simulink model "regcontrol_model_3ph_old"  (R2018b)
settings: Solver=VariableStepAuto  StartTime=0.0  StopTime=10.0  RelTol=1e-3
values from neighbouring files (symbols this model uses):
  BandWidth = Simulink.Parameter    [start.m]
  BaseVoltage = Simulink.Parameter    [start.m]
  CogenEnabled = false    [regcontrol_emulator.m]    (also in start.m = Simulink.Parameter)
  FPTphase = Simulink.Parameter(FPTphases.DEFAULT)    [regcontrol_emulator.m]    (also in start.m = 1)
  IsReversible = Simulink.Parameter    [start.m]
  LDC_Z = Simulink.Parameter    [start.m]
  MaxTap = 1.10    (= 1.1)    [Transformer.m]
  MinTap = 0.90    (= 0.9)    [Transformer.m]
  PTratio = Simulink.Parameter    [start.m]
  R = 0    [start.m]
  RevBand = Simulink.Parameter    [start.m]
  RevVreg = Simulink.Parameter    [start.m]
  TapLimitPerChange = Simulink.Parameter    [start.m]
  UsingRegulatedBus = Simulink.Parameter    [start.m]
  Vlimit = Simulink.Parameter    [start.m]
  Vreg = Simulink.Parameter    [start.m]
  X = 0    [start.m]
undefined symbols (not defined in the file or in its folder): ControlledTransformerConnection, ControlledTransformerCurrents, ControlledTransformerPowers, ControlledTransformerVoltages, ControlModes, CTRating, IsInverseTime, m, n, NumConductors, NumPhases, PresentTap, RevDelay, revLDC_Z, RevPowerThreshold, revR, revX, TapDelay, TapIncrement, TapWinding, TimeDelay, VTerminal
(part 1 of 4)
settings Model: Creator=Michael Girbino  LastModifiedBy=Michael Girbino
settings DebuggingCC: LibraryContextMissingDiagnostic=none
settings SFSimCC: SimUseLocalCustomCode=off
settings RTWCC: RTWUseLocalCustomCode=off
settings CodeAppCC: StateflowObjectComments=on

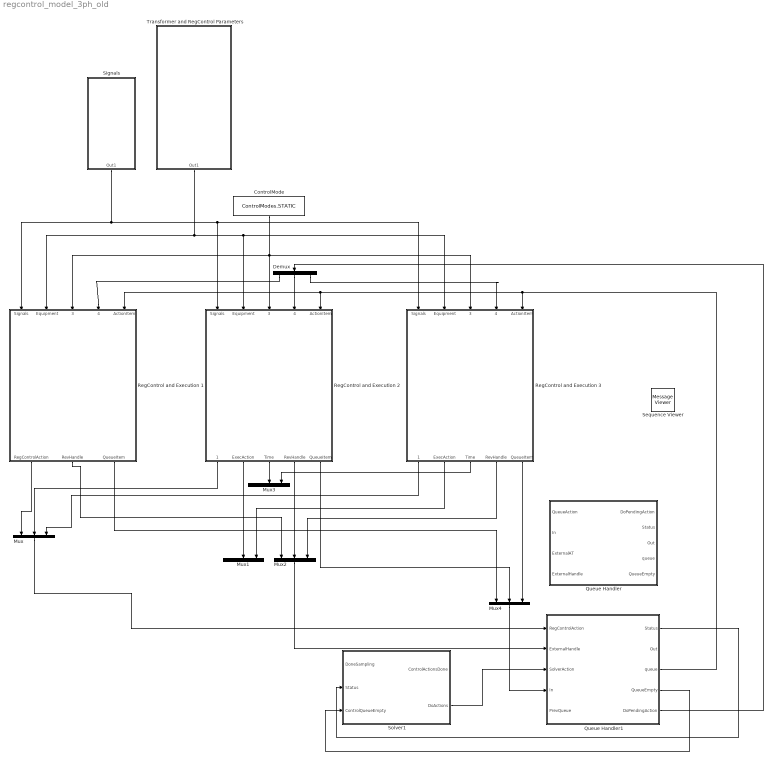
== system regcontrol_model_3ph_old ==
  ControlMode : Constant  Value=ControlModes.STATIC  OutDataTypeStr=Enum: ControlModes
  Demux : Demux  Outputs=3
  Mux{,1..4} (5 alike) : Mux  Inputs=3
  Queue Handler : Stateflow chart  TreatAsAtomicUnit=on
  Queue Handler1 : Stateflow chart  TreatAsAtomicUnit=on
  RegControl and Execution 1 : Subsystem
  RegControl and Execution 2 : Subsystem
  RegControl and Execution 3 : Subsystem
  Sequence Viewer : MessageViewer
  Signals : Subsystem
  Solver1 : Stateflow chart  TreatAsAtomicUnit=on
  Transformer and RegControl Parameters : Subsystem
  wires:
  ControlMode/1 -> RegControl and Execution 1/3(ControlMode), RegControl and Execution 3/3(ControlMode), RegControl and Execution 2/3(ControlMode)
  RegControl and Execution 1/3(QueueItem) -> Mux4/1
  Transformer and RegControl Parameters/1(Out1) -> RegControl and Execution 1/2(Equipment), RegControl and Execution 3/2(Equipment), RegControl and Execution 2/2(Equipment)
  RegControl and Execution 1/1(RegControlAction) -> Mux/1
  RegControl and Execution 1/2(RevHandle) -> Mux2/1
  Signals/1(Out1) -> RegControl and Execution 1/1(Signals), RegControl and Execution 3/1(Signals), RegControl and Execution 2/1(Signals)
  RegControl and Execution 2/1(RegControlAction) -> Mux/2
  RegControl and Execution 3/1(RegControlAction) -> Mux/3
  Mux/1 -> Queue Handler1/1(RegControlAction)
  RegControl and Execution 2/2(ExecAction) -> Mux1/2
  RegControl and Execution 3/2(ExecAction) -> Mux1/3
  RegControl and Execution 2/3(Time) -> Mux3/2
  RegControl and Execution 3/3(Time) -> Mux3/3
  RegControl and Execution 2/4(RevHandle) -> Mux2/2
  RegControl and Execution 3/4(RevHandle) -> Mux2/3
  Mux2/1 -> Queue Handler1/2(ExternalHandle)
  RegControl and Execution 2/5(QueueItem) -> Mux4/2
  RegControl and Execution 3/5(QueueItem) -> Mux4/3
  Demux/2 -> RegControl and Execution 2/4(DoPendingAction)
  Demux/1 -> RegControl and Execution 1/4(DoPendingAction)
  Demux/3 -> RegControl and Execution 3/4(DoPendingAction)
  Solver1/2(DoActions) -> Queue Handler1/3(SolverAction)
  Queue Handler1/5(DoPendingAction) -> Demux/1
  Queue Handler1/1(Status) -> Solver1/2(Status)
  Queue Handler1/3(queue) -> RegControl and Execution 1/5(ActionItem), RegControl and Execution 2/5(ActionItem), RegControl and Execution 3/5(ActionItem)
  Mux4/1 -> Queue Handler1/4(In)
  Queue Handler1/4(QueueEmpty) -> Solver1/3(ControlQueueEmpty)

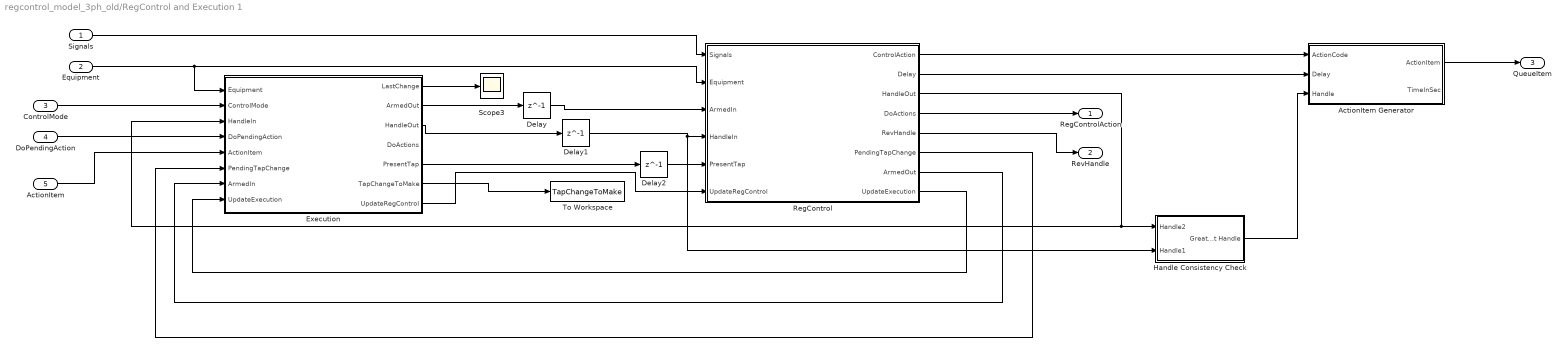
== system regcontrol_model_3ph_old/RegControl and Execution 1 ==
  Signals : Inport
  Equipment : Inport  Port=2
  ControlMode : Inport  Port=3
  DoPendingAction : Inport  Port=4
  ActionItem : Inport  Port=5
  ActionItem Generator : Subsystem
  Delay : Delay  DelayLength=1  InitialCondition=0
  Delay1 : Delay  DelayLength=1  InitialCondition=0
  Delay2 : Delay  DelayLength=1  InitialCondition=0
  Execution : Stateflow chart  TreatAsAtomicUnit=on
  Handle Consistency Check : Subsystem
  RegControl : Stateflow chart  TreatAsAtomicUnit=on
  Scope3 : Scope
  To Workspace : ToWorkspace  VariableName=TapChangeToMake  SaveFormat=Timeseries  SampleTime=-1
  RegControlAction : Outport  OutDataTypeStr=Enum: QueueActions
  RevHandle : Outport  Port=2  OutDataTypeStr=uint8
  QueueItem : Outport  Port=3  OutDataTypeStr=double  PortDimensions=[5 1]
  wires:
  RegControl/7(ArmedOut) -> Execution/7(ArmedIn)
  RegControl/6(PendingTapChange) -> Execution/6(PendingTapChange)
  Signals/1 -> RegControl/1(Signals)
  Execution/6(TapChangeToMake) -> To Workspace/1
  RegControl/3(HandleOut) -> Execution/3(HandleIn), Handle Consistency Check/1(Handle2)
  ActionItem Generator/1(ActionItem) -> QueueItem/1
  Execution/3(HandleOut) -> Delay1/1
  Handle Consistency Check/1(Greatest Handle) -> ActionItem Generator/3(Handle)
  Delay/1 -> RegControl/3(ArmedIn)
  Delay2/1 -> RegControl/5(PresentTap)
  Delay1/1 -> RegControl/4(HandleIn), Handle Consistency Check/2(Handle1)
  RegControl/2(Delay) -> ActionItem Generator/2(Delay)
  Execution/1(LastChange) -> Scope3/1
  RegControl/1(ControlAction) -> ActionItem Generator/1(ActionCode)
  Equipment/1 -> RegControl/2(Equipment), Execution/1(Equipment)
  Execution/5(PresentTap) -> Delay2/1
  RegControl/5(RevHandle) -> RevHandle/1
  Execution/2(ArmedOut) -> Delay/1
  RegControl/8(UpdateExecution) -> Execution/8(UpdateExecution)
  Execution/7(UpdateRegControl) -> RegControl/6(UpdateRegControl)
  ActionItem/1 -> Execution/5(ActionItem)
  DoPendingAction/1 -> Execution/4(DoPendingAction)
  RegControl/4(DoActions) -> RegControlAction/1
  ControlMode/1 -> Execution/2(ControlMode)

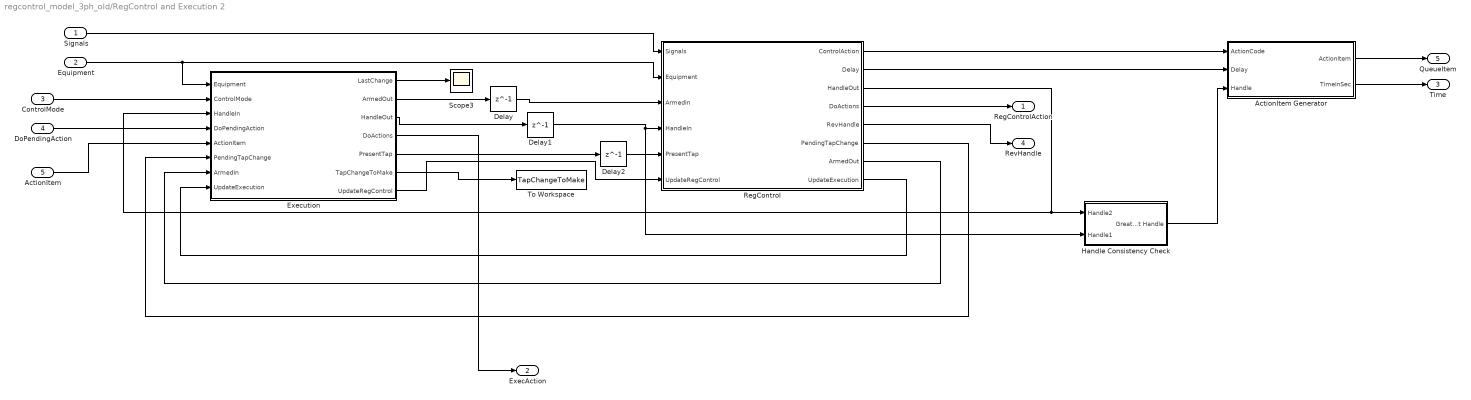
== system regcontrol_model_3ph_old/RegControl and Execution 2 ==
  Signals : Inport
  Equipment : Inport  Port=2
  ControlMode : Inport  Port=3
  DoPendingAction : Inport  Port=4
  ActionItem : Inport  Port=5
  ActionItem Generator : Subsystem
  Delay : Delay  DelayLength=1  InitialCondition=0
  Delay1 : Delay  DelayLength=1  InitialCondition=0
  Delay2 : Delay  DelayLength=1  InitialCondition=0
  Execution : Stateflow chart  TreatAsAtomicUnit=on
  Handle Consistency Check : Subsystem
  RegControl : Stateflow chart  TreatAsAtomicUnit=on
  Scope3 : Scope
  To Workspace : ToWorkspace  VariableName=TapChangeToMake  SaveFormat=Timeseries  SampleTime=-1
  RegControlAction : Outport  OutDataTypeStr=Enum: QueueActions
  ExecAction : Outport  Port=2  OutDataTypeStr=Enum: QueueActions
  Time : Outport  Port=3
  RevHandle : Outport  Port=4  OutDataTypeStr=uint8
  QueueItem : Outport  Port=5  PortDimensions=[5 1]
  wires:
  ControlMode/1 -> Execution/2(ControlMode)
  Execution/4(DoActions) -> ExecAction/1
  RegControl/4(DoActions) -> RegControlAction/1
  DoPendingAction/1 -> Execution/4(DoPendingAction)
  ActionItem Generator/2(TimeInSec) -> Time/1
  ActionItem/1 -> Execution/5(ActionItem)
  Execution/7(UpdateRegControl) -> RegControl/6(UpdateRegControl)
  RegControl/8(UpdateExecution) -> Execution/8(UpdateExecution)
  Execution/2(ArmedOut) -> Delay/1
  RegControl/5(RevHandle) -> RevHandle/1
  Execution/5(PresentTap) -> Delay2/1
  Equipment/1 -> Execution/1(Equipment), RegControl/2(Equipment)
  RegControl/1(ControlAction) -> ActionItem Generator/1(ActionCode)
  Execution/1(LastChange) -> Scope3/1
  RegControl/2(Delay) -> ActionItem Generator/2(Delay)
  Delay1/1 -> Handle Consistency Check/2(Handle1), RegControl/4(HandleIn)
  Delay2/1 -> RegControl/5(PresentTap)
  Delay/1 -> RegControl/3(ArmedIn)
  Handle Consistency Check/1(Greatest Handle) -> ActionItem Generator/3(Handle)
  Execution/3(HandleOut) -> Delay1/1
  ActionItem Generator/1(ActionItem) -> QueueItem/1
  RegControl/3(HandleOut) -> Handle Consistency Check/1(Handle2), Execution/3(HandleIn)
  Execution/6(TapChangeToMake) -> To Workspace/1
  Signals/1 -> RegControl/1(Signals)
  RegControl/6(PendingTapChange) -> Execution/6(PendingTapChange)
  RegControl/7(ArmedOut) -> Execution/7(ArmedIn)

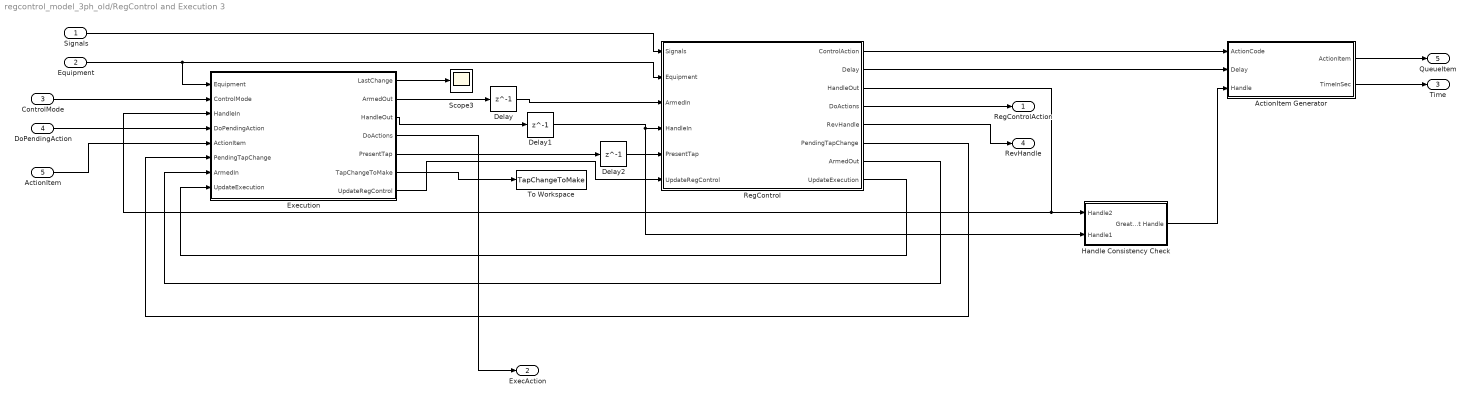
== system regcontrol_model_3ph_old/RegControl and Execution 3 ==
  Signals : Inport
  Equipment : Inport  Port=2
  ControlMode : Inport  Port=3
  DoPendingAction : Inport  Port=4
  ActionItem : Inport  Port=5
  ActionItem Generator : Subsystem
  Delay : Delay  DelayLength=1  InitialCondition=0
  Delay1 : Delay  DelayLength=1  InitialCondition=0
  Delay2 : Delay  DelayLength=1  InitialCondition=0
  Execution : Stateflow chart  TreatAsAtomicUnit=on
  Handle Consistency Check : Subsystem
  RegControl : Stateflow chart  TreatAsAtomicUnit=on
  Scope3 : Scope
  To Workspace : ToWorkspace  VariableName=TapChangeToMake  SaveFormat=Timeseries  SampleTime=-1
  RegControlAction : Outport  OutDataTypeStr=Enum: QueueActions
  ExecAction : Outport  Port=2  OutDataTypeStr=Enum: QueueActions
  Time : Outport  Port=3
  RevHandle : Outport  Port=4  OutDataTypeStr=uint8
  QueueItem : Outport  Port=5  OutDataTypeStr=double  PortDimensions=[5 1]
  wires:
  RegControl/7(ArmedOut) -> Execution/7(ArmedIn)
  RegControl/6(PendingTapChange) -> Execution/6(PendingTapChange)
  Signals/1 -> RegControl/1(Signals)
  Execution/6(TapChangeToMake) -> To Workspace/1
  RegControl/3(HandleOut) -> Execution/3(HandleIn), Handle Consistency Check/1(Handle2)
  ActionItem Generator/1(ActionItem) -> QueueItem/1
  Execution/3(HandleOut) -> Delay1/1
  Handle Consistency Check/1(Greatest Handle) -> ActionItem Generator/3(Handle)
  Delay/1 -> RegControl/3(ArmedIn)
  Delay2/1 -> RegControl/5(PresentTap)
  Delay1/1 -> RegControl/4(HandleIn), Handle Consistency Check/2(Handle1)
  RegControl/2(Delay) -> ActionItem Generator/2(Delay)
  Execution/1(LastChange) -> Scope3/1
  RegControl/1(ControlAction) -> ActionItem Generator/1(ActionCode)
  Equipment/1 -> RegControl/2(Equipment), Execution/1(Equipment)
  Execution/5(PresentTap) -> Delay2/1
  RegControl/5(RevHandle) -> RevHandle/1
  Execution/2(ArmedOut) -> Delay/1
  RegControl/8(UpdateExecution) -> Execution/8(UpdateExecution)
  Execution/7(UpdateRegControl) -> RegControl/6(UpdateRegControl)
  ActionItem/1 -> Execution/5(ActionItem)
  ActionItem Generator/2(TimeInSec) -> Time/1
  DoPendingAction/1 -> Execution/4(DoPendingAction)
  RegControl/4(DoActions) -> RegControlAction/1
  Execution/4(DoActions) -> ExecAction/1
  ControlMode/1 -> Execution/2(ControlMode)

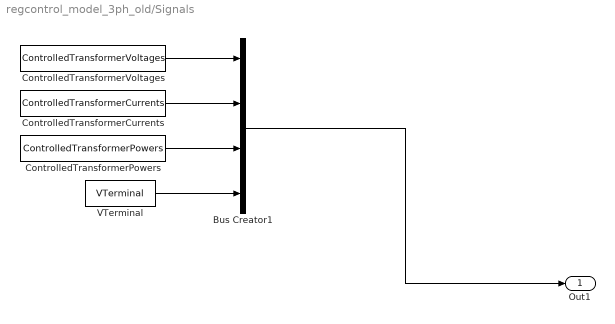
== system regcontrol_model_3ph_old/Signals ==
  Bus Creator1 : BusCreator  Inputs=4  OutDataTypeStr=Bus: SignalBus
      settings: InheritFromInputs=off
  ControlledTransformerCurrents : Constant  Value=ControlledTransformerCurrents
  ControlledTransformerPowers : Constant  Value=ControlledTransformerPowers
  ControlledTransformerVoltages : Constant  Value=ControlledTransformerVoltages
  VTerminal : Constant  Value=VTerminal
  Out1 : Outport
  wires:
  ControlledTransformerVoltages/1 -> Bus Creator1/1
  VTerminal/1 -> Bus Creator1/4
  ControlledTransformerCurrents/1 -> Bus Creator1/2
  Bus Creator1/1 -> Out1/1
  ControlledTransformerPowers/1 -> Bus Creator1/3

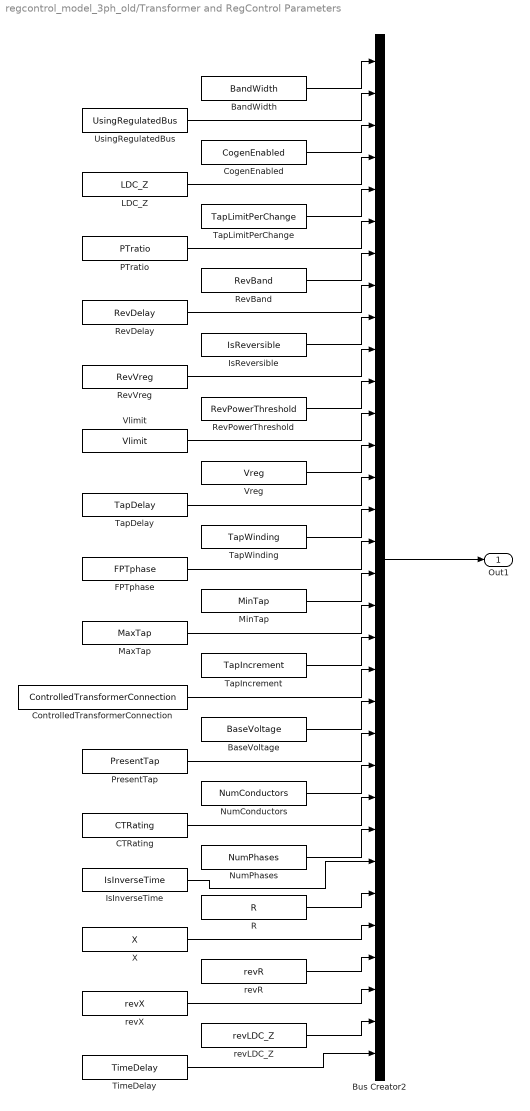
== system regcontrol_model_3ph_old/Transformer and RegControl Parameters ==
  BandWidth : Constant  Value=BandWidth
  BaseVoltage : Constant  Value=BaseVoltage
  Bus Creator2 : BusCreator  Inputs=32  OutDataTypeStr=Bus: EquipmentBus
      settings: InheritFromInputs=off
  CTRating : Constant  Value=CTRating
  CogenEnabled : Constant  Value=CogenEnabled
  ControlledTransformerConnection : Constant  Value=ControlledTransformerConnection
  FPTphase : Constant  Value=FPTphase
  IsInverseTime : Constant  Value=IsInverseTime
  IsReversible : Constant  Value=IsReversible
  LDC_Z : Constant  Value=LDC_Z
  MaxTap : Constant  Value=MaxTap
  MinTap : Constant  Value=MinTap
  NumConductors : Constant  Value=NumConductors
  NumPhases : Constant  Value=NumPhases
  PTratio : Constant  Value=PTratio
  PresentTap : Constant  Value=PresentTap
  R : Constant  Value=R
  RevBand : Constant  Value=RevBand
  RevDelay : Constant  Value=RevDelay
  RevPowerThreshold : Constant  Value=RevPowerThreshold
  RevVreg : Constant  Value=RevVreg
  TapDelay : Constant  Value=TapDelay
  TapIncrement : Constant  Value=TapIncrement
  TapLimitPerChange : Constant  Value=TapLimitPerChange
  TapWinding : Constant  Value=TapWinding
  TimeDelay : Constant  Value=TimeDelay
  UsingRegulatedBus : Constant  Value=UsingRegulatedBus
  Vlimit : Constant  Value=Vlimit
  Vreg : Constant  Value=Vreg
  X : Constant  Value=X
  revLDC_Z : Constant  Value=revLDC_Z
  revR : Constant  Value=revR
  revX : Constant  Value=revX
  Out1 : Outport
  wires:
  UsingRegulatedBus/1 -> Bus Creator2/2
  BandWidth/1 -> Bus Creator2/1
  TapWinding/1 -> Bus Creator2/15
  TapDelay/1 -> Bus Creator2/14
  Vreg/1 -> Bus Creator2/13
  Vlimit/1 -> Bus Creator2/12
  RevPowerThreshold/1 -> Bus Creator2/11
  RevVreg/1 -> Bus Creator2/10
  IsReversible/1 -> Bus Creator2/9
  RevDelay/1 -> Bus Creator2/8
  RevBand/1 -> Bus Creator2/7
  PTratio/1 -> Bus Creator2/6
  TapLimitPerChange/1 -> Bus Creator2/5
  LDC_Z/1 -> Bus Creator2/4
  CogenEnabled/1 -> Bus Creator2/3
  Bus Creator2/1 -> Out1/1
  FPTphase/1 -> Bus Creator2/16
  MinTap/1 -> Bus Creator2/17
  MaxTap/1 -> Bus Creator2/18
  TapIncrement/1 -> Bus Creator2/19
  ControlledTransformerConnection/1 -> Bus Creator2/20
  BaseVoltage/1 -> Bus Creator2/21
  PresentTap/1 -> Bus Creator2/22
  NumConductors/1 -> Bus Creator2/23
  CTRating/1 -> Bus Creator2/24
  NumPhases/1 -> Bus Creator2/25
  revLDC_Z/1 -> Bus Creator2/31
  revX/1 -> Bus Creator2/30
  revR/1 -> Bus Creator2/29
  X/1 -> Bus Creator2/28
  R/1 -> Bus Creator2/27
  IsInverseTime/1 -> Bus Creator2/26
  TimeDelay/1 -> Bus Creator2/32

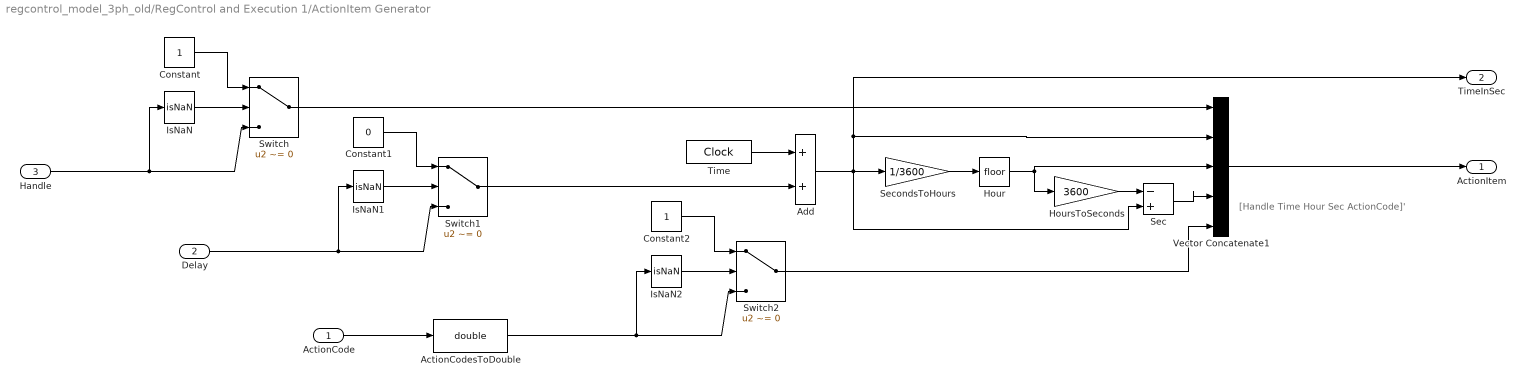
== system regcontrol_model_3ph_old/RegControl and Execution 1/ActionItem Generator ==
  note: [Handle Time Hour Sec ActionCode]'
  ActionCode : Inport
  Delay : Inport  Port=2
  Handle : Inport  Port=3
  ActionCodesToDouble : DataTypeConversion  OutDataTypeStr=double
  Add : Sum
  Constant : Constant
  Constant1 : Constant  Value=0
  Constant2 : Constant
  Hour : Rounding
  HoursToSeconds : Gain  Gain=3600
  IsNaN : RelationalOperator  Operator=isNaN  OutDataTypeStr=boolean  RndMeth=Simplest
  IsNaN1 : RelationalOperator  Operator=isNaN  OutDataTypeStr=boolean  RndMeth=Simplest
  IsNaN2 : RelationalOperator  Operator=isNaN  OutDataTypeStr=boolean  RndMeth=Simplest
  Sec : Sum  Inputs=-+
  SecondsToHours : Gain  Gain=1/3600
  Switch : Switch  Criteria=u2 ~= 0
  Switch1 : Switch  Criteria=u2 ~= 0
  Switch2 : Switch  Criteria=u2 ~= 0
  Time : DigitalClock
  Vector Concatenate1 : Concatenate  NumInputs=5
  ActionItem : Outport
  TimeInSec : Outport  Port=2
  wires:
  Add/1 -> Sec/2, SecondsToHours/1, TimeInSec/1, Vector Concatenate1/2
  Hour/1 -> Vector Concatenate1/3, HoursToSeconds/1
  SecondsToHours/1 -> Hour/1
  Vector Concatenate1/1 -> ActionItem/1
  HoursToSeconds/1 -> Sec/1
  Handle/1 -> Switch/3, IsNaN/1
  Sec/1 -> Vector Concatenate1/4
  Time/1 -> Add/1
  ActionCode/1 -> ActionCodesToDouble/1
  IsNaN/1 -> Switch/2
  Constant/1 -> Switch/1
  Switch/1 -> Vector Concatenate1/1
  Delay/1 -> IsNaN1/1, Switch1/3
  IsNaN1/1 -> Switch1/2
  Constant1/1 -> Switch1/1
  Switch1/1 -> Add/2
  ActionCodesToDouble/1 -> Switch2/3, IsNaN2/1
  IsNaN2/1 -> Switch2/2
  Constant2/1 -> Switch2/1
  Switch2/1 -> Vector Concatenate1/5

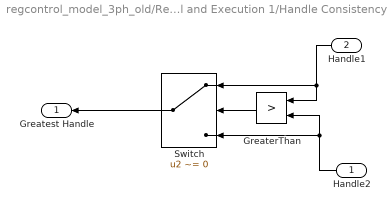
== system regcontrol_model_3ph_old/RegControl and Execution 1/Handle Consistency Check ==
  Handle2 : Inport
  Handle1 : Inport  Port=2
  GreaterThan : RelationalOperator  Operator=>  RndMeth=Simplest
  Switch : Switch  Criteria=u2 ~= 0  OutDataTypeStr=double
  Greatest Handle : Outport
  wires:
  Handle2/1 -> GreaterThan/2, Switch/3
  GreaterThan/1 -> Switch/2
  Handle1/1 -> GreaterThan/1, Switch/1
  Switch/1 -> Greatest Handle/1

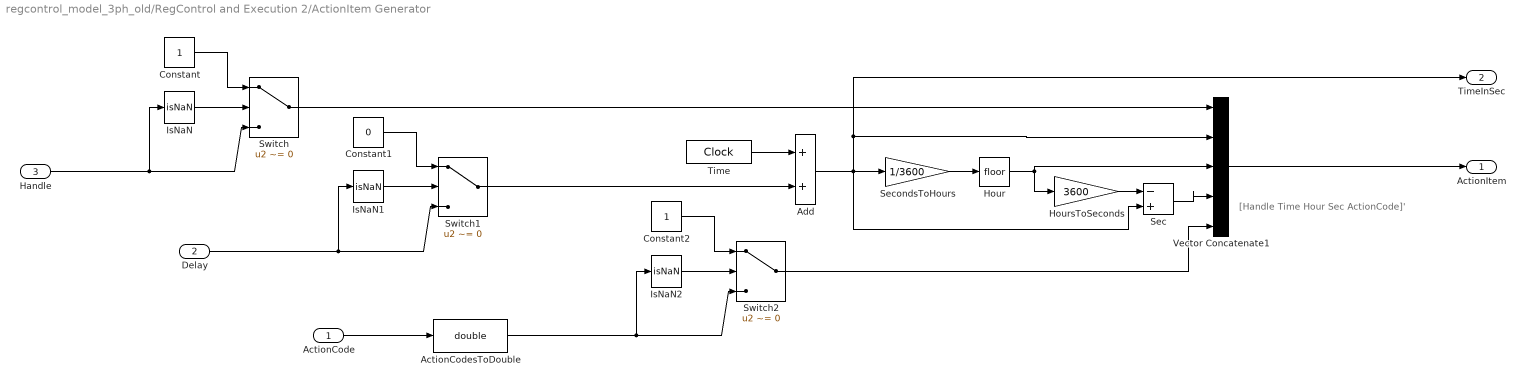
== system regcontrol_model_3ph_old/RegControl and Execution 2/ActionItem Generator ==
  note: [Handle Time Hour Sec ActionCode]'
  ActionCode : Inport
  Delay : Inport  Port=2
  Handle : Inport  Port=3
  ActionCodesToDouble : DataTypeConversion  OutDataTypeStr=double
  Add : Sum
  Constant : Constant
  Constant1 : Constant  Value=0
  Constant2 : Constant
  Hour : Rounding
  HoursToSeconds : Gain  Gain=3600
  IsNaN : RelationalOperator  Operator=isNaN  OutDataTypeStr=boolean  RndMeth=Simplest
  IsNaN1 : RelationalOperator  Operator=isNaN  OutDataTypeStr=boolean  RndMeth=Simplest
  IsNaN2 : RelationalOperator  Operator=isNaN  OutDataTypeStr=boolean  RndMeth=Simplest
  Sec : Sum  Inputs=-+
  SecondsToHours : Gain  Gain=1/3600
  Switch : Switch  Criteria=u2 ~= 0
  Switch1 : Switch  Criteria=u2 ~= 0
  Switch2 : Switch  Criteria=u2 ~= 0
  Time : DigitalClock
  Vector Concatenate1 : Concatenate  NumInputs=5
  ActionItem : Outport
  TimeInSec : Outport  Port=2
  wires:
  Switch2/1 -> Vector Concatenate1/5
  Constant2/1 -> Switch2/1
  IsNaN2/1 -> Switch2/2
  ActionCodesToDouble/1 -> IsNaN2/1, Switch2/3
  Switch1/1 -> Add/2
  Constant1/1 -> Switch1/1
  IsNaN1/1 -> Switch1/2
  Delay/1 -> Switch1/3, IsNaN1/1
  Switch/1 -> Vector Concatenate1/1
  Constant/1 -> Switch/1
  IsNaN/1 -> Switch/2
  ActionCode/1 -> ActionCodesToDouble/1
  Time/1 -> Add/1
  Sec/1 -> Vector Concatenate1/4
  Handle/1 -> IsNaN/1, Switch/3
  HoursToSeconds/1 -> Sec/1
  Vector Concatenate1/1 -> ActionItem/1
  SecondsToHours/1 -> Hour/1
  Hour/1 -> HoursToSeconds/1, Vector Concatenate1/3
  Add/1 -> Vector Concatenate1/2, TimeInSec/1, SecondsToHours/1, Sec/2

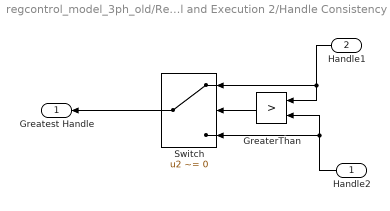
== system regcontrol_model_3ph_old/RegControl and Execution 2/Handle Consistency Check ==
  Handle2 : Inport
  Handle1 : Inport  Port=2
  GreaterThan : RelationalOperator  Operator=>  RndMeth=Simplest
  Switch : Switch  Criteria=u2 ~= 0  OutDataTypeStr=double
  Greatest Handle : Outport
  wires:
  Switch/1 -> Greatest Handle/1
  Handle1/1 -> Switch/1, GreaterThan/1
  GreaterThan/1 -> Switch/2
  Handle2/1 -> Switch/3, GreaterThan/2

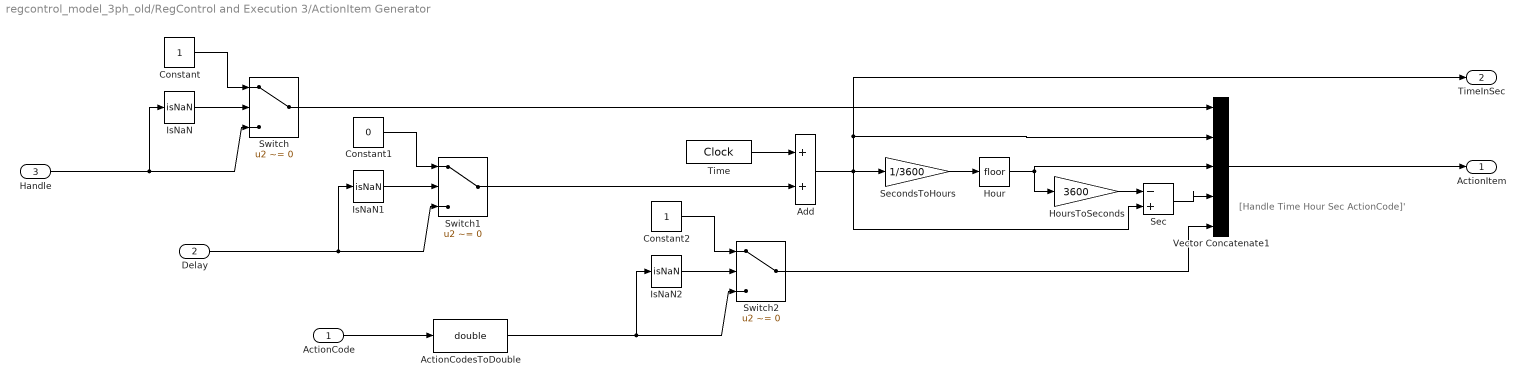
== system regcontrol_model_3ph_old/RegControl and Execution 3/ActionItem Generator ==
  note: [Handle Time Hour Sec ActionCode]'
  ActionCode : Inport
  Delay : Inport  Port=2
  Handle : Inport  Port=3
  ActionCodesToDouble : DataTypeConversion  OutDataTypeStr=double
  Add : Sum
  Constant : Constant
  Constant1 : Constant  Value=0
  Constant2 : Constant
  Hour : Rounding
  HoursToSeconds : Gain  Gain=3600
  IsNaN : RelationalOperator  Operator=isNaN  OutDataTypeStr=boolean  RndMeth=Simplest
  IsNaN1 : RelationalOperator  Operator=isNaN  OutDataTypeStr=boolean  RndMeth=Simplest
  IsNaN2 : RelationalOperator  Operator=isNaN  OutDataTypeStr=boolean  RndMeth=Simplest
  Sec : Sum  Inputs=-+
  SecondsToHours : Gain  Gain=1/3600
  Switch : Switch  Criteria=u2 ~= 0
  Switch1 : Switch  Criteria=u2 ~= 0
  Switch2 : Switch  Criteria=u2 ~= 0
  Time : DigitalClock
  Vector Concatenate1 : Concatenate  NumInputs=5
  ActionItem : Outport
  TimeInSec : Outport  Port=2
  wires:
  Add/1 -> Sec/2, SecondsToHours/1, TimeInSec/1, Vector Concatenate1/2
  Hour/1 -> Vector Concatenate1/3, HoursToSeconds/1
  SecondsToHours/1 -> Hour/1
  Vector Concatenate1/1 -> ActionItem/1
  HoursToSeconds/1 -> Sec/1
  Handle/1 -> Switch/3, IsNaN/1
  Sec/1 -> Vector Concatenate1/4
  Time/1 -> Add/1
  ActionCode/1 -> ActionCodesToDouble/1
  IsNaN/1 -> Switch/2
  Constant/1 -> Switch/1
  Switch/1 -> Vector Concatenate1/1
  Delay/1 -> IsNaN1/1, Switch1/3
  IsNaN1/1 -> Switch1/2
  Constant1/1 -> Switch1/1
  Switch1/1 -> Add/2
  ActionCodesToDouble/1 -> Switch2/3, IsNaN2/1
  IsNaN2/1 -> Switch2/2
  Constant2/1 -> Switch2/1
  Switch2/1 -> Vector Concatenate1/5

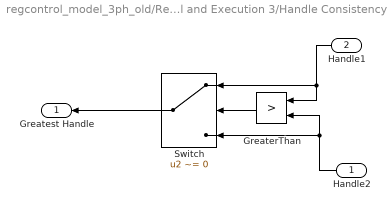
== system regcontrol_model_3ph_old/RegControl and Execution 3/Handle Consistency Check ==
  Handle2 : Inport
  Handle1 : Inport  Port=2
  GreaterThan : RelationalOperator  Operator=>  RndMeth=Simplest
  Switch : Switch  Criteria=u2 ~= 0  OutDataTypeStr=double
  Greatest Handle : Outport
  wires:
  Handle2/1 -> GreaterThan/2, Switch/3
  GreaterThan/1 -> Switch/2
  Handle1/1 -> GreaterThan/1, Switch/1
  Switch/1 -> Greatest Handle/1

== stateflow chart regcontrol_model_3ph_old/RegControl and Execution 1/Execution ==
  settings: executeAtInitialization=1
  state Push(CodeVal, DelayVal) [function]
    (default) -> (junction 341) : {ActionCode = CodeVal;
        | Delay = DelayVal;
        | HandleOut = HandleOut + 1;
        | UpdateRegControl.data = ...
        | UpdateActions.HANDLE;
        | send(UpdateRegControl);
        | DoActions.data = QueueActions.PUSH;
        | send(DoActions);}
  state UpdateLocals [parallel]
    settings: executionOrder=2
    state Asleep
      ex: UPDATED = false;
    state UpdateArmed
      en: ArmedOut = ArmedIn;
      ex: UPDATED = true;
    state UpdateHandle
      en:
      if HandleIn > HandleOut
      HandleOut = HandleIn;
      end
      ex: UPDATED = true;
    state UpdatePendingTapChange
      en: LocalPendingTapChange = ...
      PendingTapChange;
      ex: UPDATED = true;
    (default) -> UpdateLocals.Asleep
    UpdateLocals.Asleep -> UpdateHandle [order 3] : UpdateExecution[UpdateExecution.data == ...
        | UpdateActions.HANDLE]
    UpdateLocals.Asleep -> UpdatePendingTapChange [order 1] : UpdateExecution[UpdateExecution.data == ...
        | UpdateActions.PENDING_TAPCHANGE]
    UpdatePendingTapChange -> UpdateLocals.Asleep : [UPDATED]
    UpdateHandle -> UpdateLocals.Asleep : [UPDATED]
    UpdateLocals.Asleep -> UpdateArmed [order 2] : UpdateExecution[UpdateExecution.data == ...
        | UpdateActions.ARMED]
    UpdateArmed -> UpdateLocals.Asleep : [UPDATED]
  state ControlFlow [parallel]
    settings: executionOrder=1
    state Asleep
      ex: AssignInputsToLocals();
      ResetTransitionFlags();
    state MakingTapChange
      state StaticTapChange
        (default) -> (junction 165) : {TapChangeToMake = AtLeastOneTap(LocalPendingTapChange, TapIncrement);
            | % reset to no change = change - 1 program will determine if another is needed:
            | LocalPendingTapChange = 0;
            | UpdateArmed(false);}
      state EventDrivenTapChange
        (default) -> (junction 189) : {[TapChangeToMake LocalPendingTapChange] =...
            |  OneInDirectionOf(LocalPendingTapChange, TapIncrement);
            | UpdatePresentTap(TapChangeToMake);}
        (junction 189) -> (junction 190) [order 1] : [PendingTapChange ~= 0]
        (junction 189) -> (junction 191) [order 2] : {UpdateArmed(false);}
        (junction 190) -> (junction 192) : {Push(ActionCodes.ACTION_TAPCHANGE, TapDelay);}
        (junction 192) -> (junction 191)
      state TimeDrivenTapChange
        (default) -> (junction 200) : {[TapChangeToMake LocalPendingTapChange] =...
            |  OneInDirectionOf(LocalPendingTapChange, TapIncrement);
            | UpdatePresentTap(TapChangeToMake);}
        (junction 200) -> (junction 202) [order 1] : [LocalPendingTapChange ~= 0]
        (junction 200) -> (junction 203) [order 2] : {UpdateArmed(false);}
        (junction 202) -> (junction 201) : {Push(ActionCodes.ACTION_TAPCHANGE, TapDelay);}
        (junction 201) -> (junction 203)
      state MultiRateTapChange
        (default) -> (junction 210) : {[TapChangeToMake, LocalPendingTapChange] =...
            |  OneInDirectionOf(LocalPendingTapChange, TapIncrement);
            | UpdatePresentTap(TapChangeToMake);}
        (junction 210) -> (junction 212) [order 1] : [LocalPendingTapChange ~= 0]
        (junction 210) -> (junction 213) [order 2] : {UpdateArmed(false);}
        (junction 212) -> (junction 211) : {Push(ActionCodes.ACTION_TAPCHANGE, TapDelay);}
        (junction 211) -> (junction 213)
      state Finished
        en: EXIT_TAPCHANGE = true;
      (default) -> (junction 132)
      (junction 132) -> (junction 133) [order 1] : % Check to make sure control has not reset:
          | [LocalPendingTapChange == 0]
      (junction 132) -> (junction 163) [order 2]
      (junction 133) -> (junction 135) : {UpdateArmed(false);}
      (junction 163) -> StaticTapChange [order 1] : [ControlMode == ControlModes.STATIC]
      (junction 163) -> (junction 167) [order 2]
      StaticTapChange -> (junction 170)
      (junction 167) -> EventDrivenTapChange [order 1] : [ControlMode == ControlModes.EVENTDRIVEN]
      (junction 167) -> (junction 171) [order 2]
      EventDrivenTapChange -> (junction 169)
      (junction 169) -> (junction 170)
      (junction 170) -> (junction 174)
      (junction 171) -> TimeDrivenTapChange [order 1] : [ControlMode == ControlModes.TIMEDRIVEN]
      (junction 171) -> (junction 175) [order 2]
      TimeDrivenTapChange -> (junction 173)
      (junction 173) -> (junction 174)
      (junction 174) -> (junction 178)
      (junction 175) -> MultiRateTapChange [order 1] : [ControlMode == ControlModes.MULTIRATE]
      (junction 175) -> (junction 179) [order 2]
      (junction 178) -> (junction 180)
      MultiRateTapChange -> (junction 357)
      (junction 357) -> (junction 179)
      (junction 180) -> (junction 357)
      (junction 179) -> ControlFlow.MakingTapChange.Finished
      (junction 135) -> ControlFlow.MakingTapChange.Finished
    state Reversing
      state FlipCogen
        (default) -> (junction 252)
        (junction 252) -> (junction 253) [order 1] : [InCogenMode]
        (junction 252) -> (junction 254) [order 2] : {InCogenMode = true;}
        (junction 253) -> (junction 255) : {InCogenMode = false;}
        (junction 255) -> (junction 254)
      state FlipReverse
        (default) -> (junction 263)
        (junction 263) -> (junction 264) [order 1] : [InReverseMode]
        (junction 263) -> (junction 265) [order 2] : {InReverseMode = true;}
        (junction 264) -> (junction 266) : {InReverseMode = false;}
        (junction 266) -> (junction 265)
      state Finished
        en: EXIT_REVERSE = true;
      (default) -> (junction 229)
      (junction 229) -> (junction 230) [order 1] : [ReversePending]
      (junction 229) -> (junction 231) [order 2]
      (junction 230) -> (junction 242)
      (junction 242) -> (junction 238) [order 1] : [CogenEnabled]
      (junction 242) -> FlipReverse [order 2]
      (junction 238) -> FlipCogen : % Cogen mode takes precedence if present
      FlipCogen -> (junction 245)
      FlipReverse -> (junction 240)
      (junction 245) -> (junction 240)
      (junction 240) -> (junction 232) : {ReversePending = false;}
      (junction 232) -> (junction 231)
      (junction 231) -> ControlFlow.Reversing.Finished
    state Finished
    (default) -> ControlFlow.Asleep
    ControlFlow.Finished -> ControlFlow.Asleep
    ControlFlow.Asleep -> (junction 115) : DoPendingAction
    (junction 115) -> MakingTapChange [order 1] : [Code == ActionCodes.ACTION_TAPCHANGE]
    (junction 115) -> (junction 119) [order 2]
    MakingTapChange -> (junction 117) : [EXIT_TAPCHANGE]
    (junction 117) -> (junction 118)
    (junction 118) -> (junction 122)
    (junction 119) -> Reversing [order 1] : [Code == ActionCodes.ACTION_REVERSE]
    (junction 119) -> (junction 123) [order 2]
    Reversing -> (junction 122)
    (junction 122) -> (junction 124) : [EXIT_REVERSE]
    (junction 124) -> (junction 123)
    (junction 123) -> ControlFlow.Finished
  state AssignInputsToLocals [function]
    note: TapWinding
        | TapIncrement
        | TapDelay
        | CogenEnabled
    (default) -> (junction 375) : {% From Script:
        | TapWinding = Equipment.TapWinding;
        | TapIncrement = Equipment.TapIncrement;
        | TapDelay = Equipment.TapDelay;
        | CogenEnabled = Equipment.CogenEnabled;
        | PresentTap = Equipment.PresentTap;
        | TapLimitPerChange = Equipment.TapLimitPerChange;
        | % From the ControlQueue:
        | Code = ...
        | uint8(ActionItem(NewCtrlQueueFields.ActionCode));
        | % PendingTapChange:
        | % LocalPendingTapChange = PendingTapChange;
        | %ArmedOut = ArmedIn;
        | }
  state ChangeToMake = AtLeastOneTap(ProposedChange, Increment) [function]
    note: Called in STATIC mode
        | Changes 70% of the way but at least one tap, subject to maximum allowable tap change
    (default) -> (junction 283) : {NumTaps = floor(0.7 * abs(ProposedChange)/Increment);}
    (junction 283) -> (junction 284) [order 1] : [NumTaps == 0]
    (junction 283) -> (junction 285) [order 2]
    (junction 284) -> (junction 286) : {NumTaps = 1.0;} % At least 1 tap
    (junction 286) -> (junction 285)
    (junction 285) -> (junction 293)
    (junction 293) -> (junction 290) [order 1] : [NumTaps > TapLimitPerChange]
    (junction 293) -> (junction 294) [order 2]
    (junction 290) -> (junction 295) : {NumTaps = double(TapLimitPerChange);} % Bound by maximum
    (junction 295) -> (junction 294)
    (junction 294) -> (junction 302) : {LastChange = NumTaps;}
    (junction 302) -> (junction 303) [order 1] : % Check sign on change:
        | [ProposedChange > 0]
    (junction 302) -> (junction 304) [order 2] : {ChangeToMake = -1*double(NumTaps)*Increment;
        | LastChange = -1*NumTaps;}
    (junction 303) -> (junction 305) : {ChangeToMake =...
        |  double(NumTaps)*Increment;}
    (junction 305) -> (junction 304)
    (junction 304) -> (junction 306)
  state ResetTransitionFlags [function]
    (default) -> (junction 377) : {EXIT_TAPCHANGE = false;
        | EXIT_REVERSE = false;}
  state [ChangeToMake, NewProposedChange] = OneInDirectionOf(ProposedChange, Increment) [function]
    note: Computes the amount of one tap change in the direction of the pending tapchange
        | Automatically decrements the proposed change by that amount
    (default) -> (junction 318) : {LastChange = 0;}
    (junction 318) -> (junction 319) [order 1] : [ProposedChange > 0]
    (junction 318) -> (junction 320) [order 2] : {ChangeToMake = -1*Increment;
        | LastChange = -1;
        | NewProposedChange = ProposedChange + Increment;}
    (junction 319) -> (junction 321) : {ChangeToMake = Increment;
        | LastChange = 1;
        | NewProposedChange =...
        |  ProposedChange - Increment;}
    (junction 321) -> (junction 320)
    (junction 320) -> (junction 329)
    (junction 329) -> (junction 330) [order 1] : [abs(NewProposedChange) < 0.9*Increment]
    (junction 329) -> (junction 331) [order 2]
    (junction 330) -> (junction 332) : {NewProposedChange = 0;}
    (junction 332) -> (junction 331)
    (junction 331) -> (junction 333)
  state UpdatePresentTap(Change) [function]
    (default) -> (junction 415) : {
        | PresentTap = PresentTap + Change;
        | UpdateRegControl.data = ...
        | UpdateActions.PRESENT_TAP;
        | send(UpdateRegControl);
        | }
  state UpdateArmed(NewArmed) [function]
    (default) -> (junction 419) : {
        | ArmedOut = NewArmed;
        | UpdateRegControl.data = ...
        | UpdateActions.ARMED;
        | send(UpdateRegControl);
        | }
  data: CodeVal function_input; DelayVal function_input; ProposedChange function_input; Increment function_input; ChangeToMake function_output; NumTaps local double; ProposedChange function_input; Increment function_input; ChangeToMake function_output; NewProposedChange function_output; Change function_input; NewArmed function_input; Equipment input Bus: EquipmentBus; LastChange output double; ControlMode input Enum: ControlModes; HandleIn input double; ArmedOut output boolean =false; HandleOut output double =0; DoActions output Enum: QueueActions; PresentTap output double; EXIT_REVERSE local boolean; InReverseMode local boolean; EXIT_TAPCHANGE local boolean; ReversePending local boolean; InCogenMode local boolean; DoPendingAction input boolean; TapWinding local uint8; TapIncrement local double; TapDelay local double; CogenEnabled local boolean =false; Code local uint8; ActionItem input double size=[1 5]; TapChangeToMake output double; PendingTapChange input double size=[1]; LocalPendingTapChange local double =double(0); ArmedIn input boolean; TapLimitPerChange local uint8 =uint8(16); UpdateRegControl output Enum: UpdateActions; UpdateExecution input Enum: UpdateActions; UPDATED local boolean =false

== stateflow chart regcontrol_model_3ph_old/RegControl and Execution 2/Execution ==
  settings: executeAtInitialization=1
  state Push(CodeVal, DelayVal) [function]
    (default) -> (junction 341) : {ActionCode = CodeVal;
        | Delay = DelayVal;
        | HandleOut = HandleOut + 1;
        | UpdateRegControl.data = ...
        | UpdateActions.HANDLE;
        | send(UpdateRegControl);
        | DoActions.data = QueueActions.PUSH;
        | send(DoActions);}
  state UpdateLocals [parallel]
    settings: executionOrder=2
    state Asleep
      ex: UPDATED = false;
    state UpdateArmed
      en: ArmedOut = ArmedIn;
      ex: UPDATED = true;
    state UpdateHandle
      en:
      if HandleIn > HandleOut
      HandleOut = HandleIn;
      end
      ex: UPDATED = true;
    state UpdatePendingTapChange
      en: LocalPendingTapChange = ...
      PendingTapChange;
      ex: UPDATED = true;
    (default) -> UpdateLocals.Asleep
    UpdateLocals.Asleep -> UpdateHandle [order 3] : UpdateExecution[UpdateExecution.data == ...
        | UpdateActions.HANDLE]
    UpdateLocals.Asleep -> UpdatePendingTapChange [order 1] : UpdateExecution[UpdateExecution.data == ...
        | UpdateActions.PENDING_TAPCHANGE]
    UpdatePendingTapChange -> UpdateLocals.Asleep : [UPDATED]
    UpdateHandle -> UpdateLocals.Asleep : [UPDATED]
    UpdateLocals.Asleep -> UpdateArmed [order 2] : UpdateExecution[UpdateExecution.data == ...
        | UpdateActions.ARMED]
    UpdateArmed -> UpdateLocals.Asleep : [UPDATED]
  state ControlFlow [parallel]
    settings: executionOrder=1
    state Asleep
      ex: AssignInputsToLocals();
      ResetTransitionFlags();
    state MakingTapChange
      state StaticTapChange
        (default) -> (junction 165) : {TapChangeToMake = AtLeastOneTap(LocalPendingTapChange, TapIncrement);
            | % reset to no change = change - 1 program will determine if another is needed:
            | LocalPendingTapChange = 0;
            | UpdateArmed(false);}
      state EventDrivenTapChange
        (default) -> (junction 189) : {[TapChangeToMake LocalPendingTapChange] =...
            |  OneInDirectionOf(LocalPendingTapChange, TapIncrement);
            | UpdatePresentTap(TapChangeToMake);}
        (junction 189) -> (junction 190) [order 1] : [PendingTapChange ~= 0]
        (junction 189) -> (junction 191) [order 2] : {UpdateArmed(false);}
        (junction 190) -> (junction 192) : {Push(ActionCodes.ACTION_TAPCHANGE, TapDelay);}
        (junction 192) -> (junction 191)
      state TimeDrivenTapChange
        (default) -> (junction 200) : {[TapChangeToMake LocalPendingTapChange] =...
            |  OneInDirectionOf(LocalPendingTapChange, TapIncrement);
            | UpdatePresentTap(TapChangeToMake);}
        (junction 200) -> (junction 202) [order 1] : [LocalPendingTapChange ~= 0]
        (junction 200) -> (junction 203) [order 2] : {UpdateArmed(false);}
        (junction 202) -> (junction 201) : {Push(ActionCodes.ACTION_TAPCHANGE, TapDelay);}
        (junction 201) -> (junction 203)
      state MultiRateTapChange
        (default) -> (junction 210) : {[TapChangeToMake, LocalPendingTapChange] =...
            |  OneInDirectionOf(LocalPendingTapChange, TapIncrement);
            | UpdatePresentTap(TapChangeToMake);}
        (junction 210) -> (junction 212) [order 1] : [LocalPendingTapChange ~= 0]
        (junction 210) -> (junction 213) [order 2] : {UpdateArmed(false);}
        (junction 212) -> (junction 211) : {Push(ActionCodes.ACTION_TAPCHANGE, TapDelay);}
        (junction 211) -> (junction 213)
      state Finished
        en: EXIT_TAPCHANGE = true;
      (default) -> (junction 132)
      (junction 132) -> (junction 133) [order 1] : % Check to make sure control has not reset:
          | [LocalPendingTapChange == 0]
      (junction 132) -> (junction 163) [order 2]
      (junction 133) -> (junction 135) : {UpdateArmed(false);}
      (junction 163) -> StaticTapChange [order 1] : [ControlMode == ControlModes.STATIC]
      (junction 163) -> (junction 167) [order 2]
      StaticTapChange -> (junction 170)
      (junction 167) -> EventDrivenTapChange [order 1] : [ControlMode == ControlModes.EVENTDRIVEN]
      (junction 167) -> (junction 171) [order 2]
      EventDrivenTapChange -> (junction 169)
      (junction 169) -> (junction 170)
      (junction 170) -> (junction 174)
      (junction 171) -> TimeDrivenTapChange [order 1] : [ControlMode == ControlModes.TIMEDRIVEN]
      (junction 171) -> (junction 175) [order 2]
      TimeDrivenTapChange -> (junction 173)
      (junction 173) -> (junction 174)
      (junction 174) -> (junction 178)
      (junction 175) -> MultiRateTapChange [order 1] : [ControlMode == ControlModes.MULTIRATE]
      (junction 175) -> (junction 179) [order 2]
      (junction 178) -> (junction 180)
      MultiRateTapChange -> (junction 357)
      (junction 357) -> (junction 179)
      (junction 180) -> (junction 357)
      (junction 179) -> ControlFlow.MakingTapChange.Finished
      (junction 135) -> ControlFlow.MakingTapChange.Finished
    state Reversing
      state FlipCogen
        (default) -> (junction 252)
        (junction 252) -> (junction 253) [order 1] : [InCogenMode]
        (junction 252) -> (junction 254) [order 2] : {InCogenMode = true;}
        (junction 253) -> (junction 255) : {InCogenMode = false;}
        (junction 255) -> (junction 254)
      state FlipReverse
        (default) -> (junction 263)
        (junction 263) -> (junction 264) [order 1] : [InReverseMode]
        (junction 263) -> (junction 265) [order 2] : {InReverseMode = true;}
        (junction 264) -> (junction 266) : {InReverseMode = false;}
        (junction 266) -> (junction 265)
      state Finished
        en: EXIT_REVERSE = true;
      (default) -> (junction 229)
      (junction 229) -> (junction 230) [order 1] : [ReversePending]
      (junction 229) -> (junction 231) [order 2]
      (junction 230) -> (junction 242)
      (junction 242) -> (junction 238) [order 1] : [CogenEnabled]
      (junction 242) -> FlipReverse [order 2]
      (junction 238) -> FlipCogen : % Cogen mode takes precedence if present
      FlipCogen -> (junction 245)
      FlipReverse -> (junction 240)
      (junction 245) -> (junction 240)
      (junction 240) -> (junction 232) : {ReversePending = false;}
      (junction 232) -> (junction 231)
      (junction 231) -> ControlFlow.Reversing.Finished
    state Finished
    (default) -> ControlFlow.Asleep
    ControlFlow.Finished -> ControlFlow.Asleep
    ControlFlow.Asleep -> (junction 115) : DoPendingAction
    (junction 115) -> MakingTapChange [order 1] : [Code == ActionCodes.ACTION_TAPCHANGE]
    (junction 115) -> (junction 119) [order 2]
    MakingTapChange -> (junction 117) : [EXIT_TAPCHANGE]
    (junction 117) -> (junction 118)
    (junction 118) -> (junction 122)
    (junction 119) -> Reversing [order 1] : [Code == ActionCodes.ACTION_REVERSE]
    (junction 119) -> (junction 123) [order 2]
    Reversing -> (junction 122)
    (junction 122) -> (junction 124) : [EXIT_REVERSE]
    (junction 124) -> (junction 123)
    (junction 123) -> ControlFlow.Finished
  state AssignInputsToLocals [function]
    note: TapWinding
        | TapIncrement
        | TapDelay
        | CogenEnabled
    (default) -> (junction 375) : {% From Script:
        | TapWinding = Equipment.TapWinding;
        | TapIncrement = Equipment.TapIncrement;
        | TapDelay = Equipment.TapDelay;
        | CogenEnabled = Equipment.CogenEnabled;
        | PresentTap = Equipment.PresentTap;
        | TapLimitPerChange = Equipment.TapLimitPerChange;
        | % From the ControlQueue:
        | Code = ...
        | uint8(ActionItem(NewCtrlQueueFields.ActionCode));
        | % PendingTapChange:
        | % LocalPendingTapChange = PendingTapChange;
        | %ArmedOut = ArmedIn;
        | }
  state ChangeToMake = AtLeastOneTap(ProposedChange, Increment) [function]
    note: Called in STATIC mode
        | Changes 70% of the way but at least one tap, subject to maximum allowable tap change
    (default) -> (junction 283) : {NumTaps = floor(0.7 * abs(ProposedChange)/Increment);}
    (junction 283) -> (junction 284) [order 1] : [NumTaps == 0]
    (junction 283) -> (junction 285) [order 2]
    (junction 284) -> (junction 286) : {NumTaps = 1.0;} % At least 1 tap
    (junction 286) -> (junction 285)
    (junction 285) -> (junction 293)
    (junction 293) -> (junction 290) [order 1] : [NumTaps > TapLimitPerChange]
    (junction 293) -> (junction 294) [order 2]
    (junction 290) -> (junction 295) : {NumTaps = double(TapLimitPerChange);} % Bound by maximum
    (junction 295) -> (junction 294)
    (junction 294) -> (junction 302) : {LastChange = NumTaps;}
    (junction 302) -> (junction 303) [order 1] : % Check sign on change:
        | [ProposedChange > 0]
    (junction 302) -> (junction 304) [order 2] : {ChangeToMake = -1*double(NumTaps)*Increment;
        | LastChange = -1*NumTaps;}
    (junction 303) -> (junction 305) : {ChangeToMake =...
        |  double(NumTaps)*Increment;}
    (junction 305) -> (junction 304)
    (junction 304) -> (junction 306)
  state ResetTransitionFlags [function]
    (default) -> (junction 377) : {EXIT_TAPCHANGE = false;
        | EXIT_REVERSE = false;}
  state [ChangeToMake, NewProposedChange] = OneInDirectionOf(ProposedChange, Increment) [function]
    note: Computes the amount of one tap change in the direction of the pending tapchange
        | Automatically decrements the proposed change by that amount
    (default) -> (junction 318) : {LastChange = 0;}
    (junction 318) -> (junction 319) [order 1] : [ProposedChange > 0]
    (junction 318) -> (junction 320) [order 2] : {ChangeToMake = -1*Increment;
        | LastChange = -1;
        | NewProposedChange = ProposedChange + Increment;}
    (junction 319) -> (junction 321) : {ChangeToMake = Increment;
        | LastChange = 1;
        | NewProposedChange =...
        |  ProposedChange - Increment;}
    (junction 321) -> (junction 320)
    (junction 320) -> (junction 329)
    (junction 329) -> (junction 330) [order 1] : [abs(NewProposedChange) < 0.9*Increment]
    (junction 329) -> (junction 331) [order 2]
    (junction 330) -> (junction 332) : {NewProposedChange = 0;}
    (junction 332) -> (junction 331)
    (junction 331) -> (junction 333)
  state UpdatePresentTap(Change) [function]
    (default) -> (junction 415) : {
        | PresentTap = PresentTap + Change;
        | UpdateRegControl.data = ...
        | UpdateActions.PRESENT_TAP;
        | send(UpdateRegControl);
        | }
  state UpdateArmed(NewArmed) [function]
    (default) -> (junction 419) : {
        | ArmedOut = NewArmed;
        | UpdateRegControl.data = ...
        | UpdateActions.ARMED;
        | send(UpdateRegControl);
        | }
  data: CodeVal function_input; DelayVal function_input; ProposedChange function_input; Increment function_input; ChangeToMake function_output; NumTaps local double; ProposedChange function_input; Increment function_input; ChangeToMake function_output; NewProposedChange function_output; Change function_input; NewArmed function_input; Equipment input Bus: EquipmentBus; LastChange output double; ControlMode input Enum: ControlModes; HandleIn input double; ArmedOut output boolean =false; HandleOut output double =0; DoActions output Enum: QueueActions; PresentTap output double; EXIT_REVERSE local boolean; InReverseMode local boolean; EXIT_TAPCHANGE local boolean; ReversePending local boolean; InCogenMode local boolean; DoPendingAction input boolean; TapWinding local uint8; TapIncrement local double; TapDelay local double; CogenEnabled local boolean =false; Code local uint8; ActionItem input double size=[1 5]; TapChangeToMake output double; PendingTapChange input double size=[1]; LocalPendingTapChange local double =double(0); ArmedIn input boolean; TapLimitPerChange local uint8 =uint8(16); UpdateRegControl output Enum: UpdateActions; UpdateExecution input Enum: UpdateActions; UPDATED local boolean =false
